simulink model "motor_control_sim"  (R2020b)
settings: Solver=VariableStepAuto  StartTime=0.0  StopTime=inf  RelTol=1e-3
settings Model: Creator=nelso  LastModifiedBy=nelso

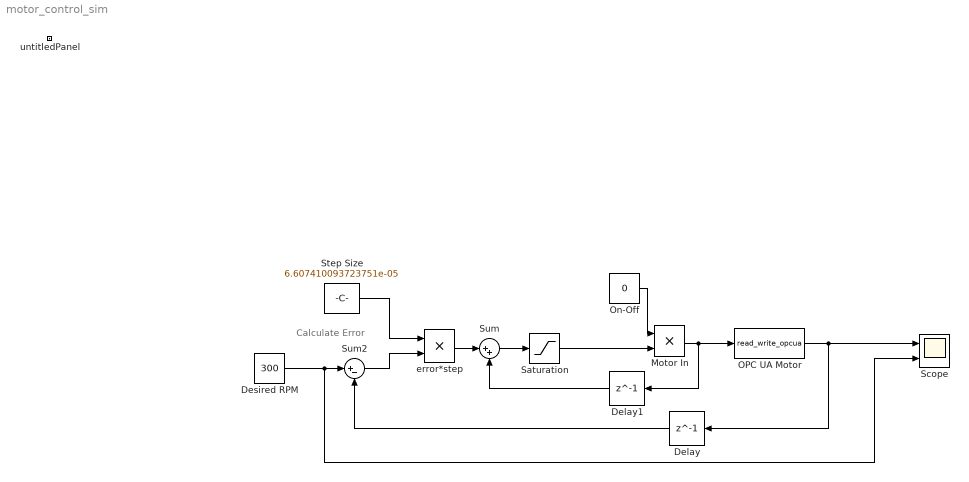
== system motor_control_sim ==
  note: Calculate Error
  Delay : Delay  DelayLength=1
  Delay1 : Delay  DelayLength=1
  Desired RPM : Constant  Value=300
  Motor In : Product
  OPC UA Motor : MATLABFcn  MATLABFcn=read_write_opcua  OutputDimensions=1  Output1D=off
  On-Off : Constant  Value=0
  Saturation : Saturate  UpperLimit=1  LowerLimit=0
  Scope : Scope  NumInputPorts=2
  Step Size : Constant  Value=6.607410093723751e-05
  Sum : Sum  Inputs=|++
  Sum2 : Sum  Inputs=|+-
  error*step : Product
  untitledPanel : Subsystem  Tag=HiddenForWebPanel  IsWebBlockPanel=on
  wires:
  OPC UA Motor/1 -> Scope/1, Delay/1
  Delay/1 -> Sum2/2
  Desired RPM/1 -> Scope/2, Sum2/1
  Sum2/1 -> error*step/2
  Step Size/1 -> error*step/1
  On-Off/1 -> Motor In/1
  Motor In/1 -> OPC UA Motor/1, Delay1/1
  error*step/1 -> Sum/1
  Delay1/1 -> Sum/2
  Sum/1 -> Saturation/1
  Saturation/1 -> Motor In/2

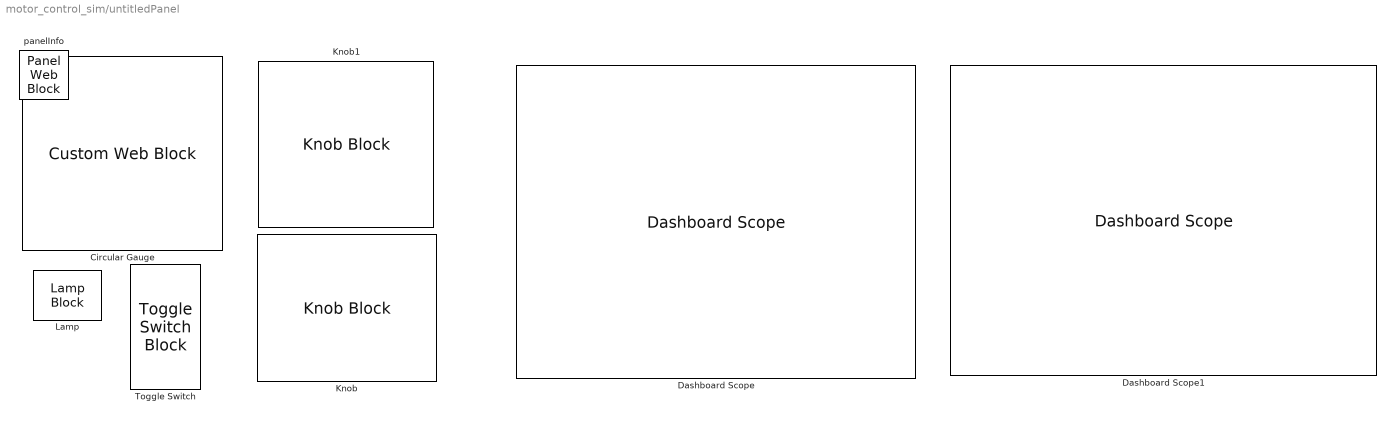
== system motor_control_sim/untitledPanel ==
  Circular Gauge : CustomWebBlock  Tag=HiddenForWebPanel  PanelInfo="{\"panelId\":\"panelId-d324ff84-3bbd-4d98-971a-cec95afe0b01\",\"type\":\"panelChild\",\"version\":\"2019b\",\"zIndex\":1500002}"  LabelPosition=Hide  ShowInitialText=on  Configuration="{\"components\":[{\"name\":\"CircularScaleComponent\",\"settings\":{\"bounds\":{\"max\":500,\"min\":0,\"tickInterval\":\"auto\"},\"direction\":\"cw\",\"flipLimits\":0,\"innerRadius\":0.75,\"internalTickHeightScaleFactor\":1,\"labelColor\":[255,252,199],\"labelFont\":{\"font\":\"Arial\",\"fontSize\":12},\"labelTransparency\":1,\"minorTickHeightScaleFactor\":0.2,\"needleImage\":{\"size\":[1890,567],\"src\":\"data:image\\/svg+xml;base64,PD94bWwgdmVyc2lvbj0iMS4wIiBlbmNvZGluZz0iVVRGLTgiIHN0YW5kYWxvbmU9Im5vIj8+CjxzdmcKICAgeG1sbnM6ZGM9Imh0dHA6Ly9wdXJsLm9yZy9kYy9lbGVtZW50cy8xLjEvIgogICB4bWxuczpjYz0iaHR0cDovL2NyZWF0aXZlY29tbW9ucy5vcmcvbnMjIgogICB4bWxuczpyZGY9Imh0dHA6Ly93d3cudzMub3JnLzE5OTkvMDIvMjItcmRmLXN5bnRheC1ucyMiCiAgIHhtbG5zOnN2Zz0iaHR0cDovL3d3dy53My5vcmcvMjAwMC9zdmciCiAgIHhtbG5zPSJodHRwOi8vd3d3LnczLm9yZy8yMDAwL3N2ZyIKICAgeG1sbnM6 ...(+4096 chars)\"},\"needleOffset\":[0.1610917094974375,0],\"needleOrientation\":-45,\"needleRotation\":180.59702388394928,\"needleSize\":{\"height\":0.13032601008944536,\"width\":0.416859542883425},\"outerRadius\":0.9,\"position\":[0.06486742424242424,0.05627705627705628,0.8917748917748918,0.8787878787878788],\"scaleAngle\":270,\"scaleAngleOffset\":135,\"scaleColors\":[],\"scaleColorsSize\":0.2,\"scalePosition\":[0,0,1,1],\"showLabels\":1,\"showMinorTicks\":1,\"showSpanLine\":1,\"showTicks\":1,\"tickColor\":[255,255,200],\"tickTransparency\":1,\"valueBarColor\":[0,114,189],\"valueBarPosition\":[0,0,1,1],\"valueBarSize\":0.2,\"valueBarTransparency\":1}},{\"name\":\"BackgroundImageComponent\",\"settings\":{\"image\":{\"size\":[500,500],\"src\":\"data:image\\/svg+xml;base64,PD94bWwgdmVyc2lvbj0iMS4wIiBlbmNvZGluZz0iVVRGLTgiIHN0YW5kYWxvbmU9Im5vIj8+CjxzdmcKICAgeG1sbnM6ZGM9Imh0dHA6Ly9wdXJsLm9yZy9kYy9lbGVtZW50cy8xLjEvIgogICB4bWxuczpjYz0iaHR0cDovL2NyZWF0aXZlY29tbW9ucy5vcmcvbnMjIgogICB4bWxuczpyZGY9Imh0dHA6Ly93d3cudzMub3JnLzE5OTkvMDIvMjItcmRmLXN5bnRheC1ucyMiCiAgIHhtbG5zOnN2Zz0iaHR0cDovL3d3dy53My5vcmcvMjAwMC9zdmciCiAgIHhtbG5zPSJodHRwOi8vd3d3LnczLm9yZy8yMDAwL3N2ZyIKICAgeG1sbnM6 ...(+9964 chars)\"},\"position\":[0,0,1,1],\"scaleMode\":\"0\"}},{\"name\":\"ForegroundImageComponent\",\"settings\":{\"image\":{\"size\":[0,0],\"src\":\"default\",\"srcOrientation\":[]},\"isForeground\":1,\"position\":[0,0,1,1],\"scaleMode\":\"0\"}}],\"settings\":{\"BindingType\":\"signal\",\"aspectRatio\":1.0309278350515463,\"direction\":\"cw\",\"fixedAspectRatio\":\"on\",\"flipLimits\":0,\"orientation\":\"horizontal\"},\"type\":\"CircularGauge\"}"
  Dashboard Scope : DashboardScope  Tag=HiddenForWebPanel  PanelInfo="{\"panelId\":\"panelId-d324ff84-3bbd-4d98-971a-cec95afe0b01\",\"type\":\"panelChild\",\"version\":\"2019b\",\"zIndex\":1500008}"  Ymin=0  Ymax=500  ScaleAtStop=off
  Dashboard Scope1 : DashboardScope  Tag=HiddenForWebPanel  PanelInfo="{\"panelId\":\"panelId-d324ff84-3bbd-4d98-971a-cec95afe0b01\",\"type\":\"panelChild\",\"version\":\"2019b\",\"zIndex\":1500018}"  Ymin=-0.1  Ymax=1.1  ScaleAtStop=off
  Knob : KnobBlock  Tag=HiddenForWebPanel  PanelInfo="{\"panelId\":\"panelId-d324ff84-3bbd-4d98-971a-cec95afe0b01\",\"type\":\"panelChild\",\"version\":\"2019b\",\"zIndex\":1500014}"  ScaleMin=100  ScaleMax=500
  Knob1 : KnobBlock  Tag=HiddenForWebPanel  PanelInfo="{\"panelId\":\"panelId-d324ff84-3bbd-4d98-971a-cec95afe0b01\",\"type\":\"panelChild\",\"version\":\"2019b\",\"zIndex\":1500016}"  ScaleMin=0.00001  ScaleMax=0.0001  TickInterval=1e-5
  Lamp : LampBlock  Tag=HiddenForWebPanel  PanelInfo="{\"panelId\":\"panelId-d324ff84-3bbd-4d98-971a-cec95afe0b01\",\"type\":\"panelChild\",\"version\":\"2019b\",\"zIndex\":1500006}"
  Toggle Switch : ToggleSwitchBlock  Tag=HiddenForWebPanel  PanelInfo="{\"panelId\":\"panelId-d324ff84-3bbd-4d98-971a-cec95afe0b01\",\"type\":\"panelChild\",\"version\":\"2019b\",\"zIndex\":1500010}"
      settings: Values={{'Off', 'On'}, [0 1]}
  panelInfo : PanelWebBlock  Tag=HiddenForWebPanel  PanelInfo="{\"compacted\":false,\"height\":377,\"labels\":{},\"left\":113,\"name\":\"untitledPanel\",\"panelId\":\"panelId-d324ff84-3bbd-4d98-971a-cec95afe0b01\",\"top\":62,\"type\":\"panel\",\"version\":\"2019b\",\"visible\":true,\"width\":1453,\"zIndex\":1500002}"
